simulink model "AMR_Testing"  (R2023b)
settings: Solver=FixedStepAuto  StartTime=0.0  StopTime=inf  FixedStep=1e-3  RelTol=1e-3
model workspace (MAT data in the model file):
  mdlWSDbList = ["C:\Users\matlab.cut\Desktop\AMR\canbus_files\tramontina_database_mobotic.dbc" "C:\Users\matlab.cut\Desktop\AMR\canbus_files\tramontina_database_nvidia.dbc" "C:\Users\matlab.cut\Desktop\AMR\canbus_files\tramontina_database_sick_modbus.dbc" "C:\Users\matlab.cut\Desktop\AMR\canbus_files\tramontina_database_xsens.dbc" "tramontina_database_curtis.dbc"]
  min_motor_rpm = 30
  vehicle_track = 877
  vehicle_wheelbase = 2367
  wheel_diameter = 360
  wheel_radius = 180
undefined symbols (not defined in the file or in its folder): Down, Pull
libraries: speedgoatlib_IO60X_IO69X x12, tramontina_database_curtislib x11, tramontina_database_nvidialib x5, simulink x4, tramontina_database_xsenslib x3, speedgoatlib_IO691 x2, simulink_extras x1, tramontina_database_sick_modbuslib x1, canmsglib x1
(part 1 of 2)
settings Model: SimulationMode=external  ExtModeEnableFloating=off  Creator=matlab.cut  LastModifiedBy=matlab.cut
settings SolverCC: ConcurrentTasks=on  PositivePriorityOrder=on
settings OptimizationCC: BlockReduction=off  OptimizeBlockIOStorage=off
settings DebuggingCC: TasksWithSamePriorityMsg=none
settings HardwareCC: ProdBitPerLong=64  ProdLongLongMode=on  ProdHWDeviceType=Intel->x86-64 (Linux 64)
settings ModelReferenceCC: ModelReferenceNumInstancesAllowed=Single
settings RTWCC: Description=Simulink Real-Time  SystemTargetFile=slrealtime.tlc  TemplateMakefile=slrealtime_default_tmf  Toolchain=Simulink Real-Time Toolchain  BuildConfiguration=Faster Runs  CodeExecutionProfiling=on  TargetLang=C++
settings CodeAppCC: MaxIdLength=127

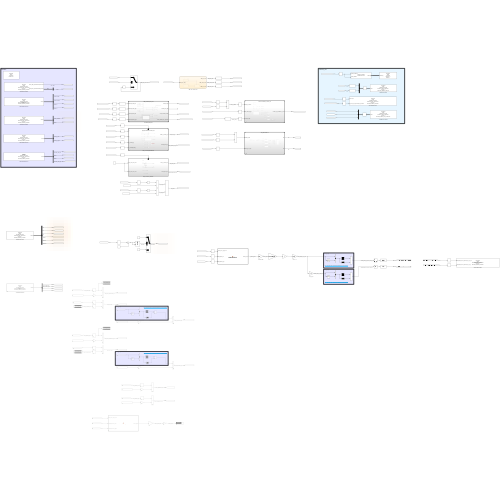
[thumbnail: Simulink's stored preview of the top-level diagram]
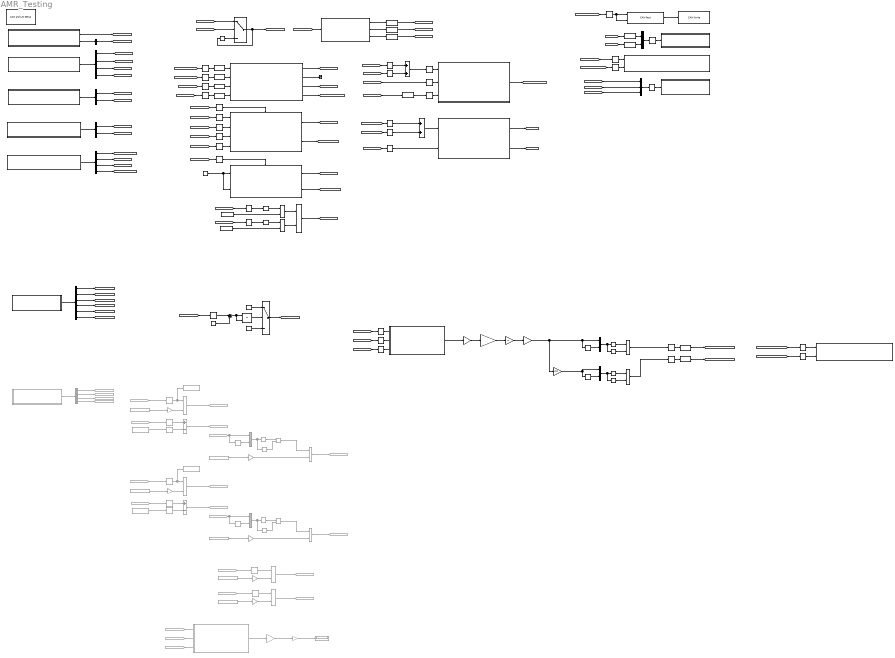
== system AMR_Testing ==
  note: moving_avg
  note: interface_out
  note: REF ->> https://www.youtube.com/watch?v=BV3H-0wlcSs&ab_channel=EmbeddedRoom
  note: REF ->> https://www.youtube.com/watch?v=BV3H-0wlcSs&ab_channel=EmbeddedRoom
  note: moving_avg
  note: REF ->> https://www.youtube.com/watch?v=BV3H-0wlcSs&ab_channel=EmbeddedRoom
  note: moving_avg
  note: REF ->> https://www.youtube.com/watch?v=BV3H-0wlcSs&ab_channel=EmbeddedRoom
  note: moving_avg
  note: interface
  AMR_ControlUnit_AutoMode : Subsystem  TreatAsAtomicUnit=on
  AMR_ControlUnit_ManualMode : ModelReference  ModelNameDialog=AMR_ManualModeControlUnit_23b.slx  SimulationMode=Normal  ModelReferenceVersion=1.27  EnablePortName=Enable  EnablePortStatesWhenEnabling=held
  AMR_oper_mode_chart : Stateflow chart  TreatAsAtomicUnit=on
  AND : Logic  AllPortsSameDT=off  OutDataTypeStr=boolean
  Abs : Abs  SaturateOnIntegerOverflow=off
  Abs3 : Abs  SaturateOnIntegerOverflow=off
  Add1 : Sum
  Add2 : Sum
  Bus Creator1 : BusCreator  Inputs=2
  Bus Creator2 : BusCreator  Inputs=3
  Bus Selector10 : BusSelector  OutputSignals=ID422_curtis_feedback_message_left.motor_rpm_left,ID423_curtis_feedback_message_right.motor_rpm_right
  Bus Selector11 : BusSelector  OutputSignals=Status  OutputAsBus=on
  Bus Selector12 : BusSelector  OutputSignals=ID368_joystick_axes.joystick_throttle,ID368_joystick_axes.joystick_direction,ID369_joystick_buttons.button_5,ID369_joystick_buttons.button_6
  Bus Selector13 : BusSelector  OutputSignals=ID1830_controller_status_left.controller_mode_left,ID1830_controller_status_left.MessageStatus.Status,ID1831_controller_status_right.MessageStatus.Status,ID1831_controller_status_right.controller_mode_right
  Bus Selector5 : BusSelector  OutputSignals=ID49_DeltaV.X,ID49_DeltaV.Y,ID49_DeltaV.Z,ID49_DeltaV.MessageStatus.Status,ID17_StatusWord.GNSSfix,ID17_StatusWord.RtkStatus
  Bus Selector6 : BusSelector  Commented=on  OutputSignals=ID934_curtis_encoder_left.rotor_position_left,ID935_curtis_encoder_right.rotor_position_rigth,ID934_curtis_encoder_left.MessageStatus.Status,ID935_curtis_encoder_right.MessageStatus.Status
  Bus Selector7 : BusSelector  Commented=on  OutputSignals=ID934_curtis_encoder_left.rotor_position_left,ID935_curtis_encoder_right.rotor_position_rigth,ID934_curtis_encoder_left.MessageStatus.Status,ID935_curtis_encoder_right.MessageStatus.Status
  Bus Selector9 : BusSelector  OutputSignals=ID288_mobotic_feedback_pos.position_feedback,ID288_mobotic_feedback_pos.MessageStatus.Status
  "CAN DB Parser Read " : Subsystem
      settings: OpenFcn=sg_can.OpenFcnRead;
      mask Help: eval('sg.utils.help.show(''io_main/refentry_ref_can_ofa_parsing_read'');')
      mask Display: disp('Speedgoat\nIO691\nCAN DB Parser Read\nModule ID: IO691 - Module ID 1\nChannel:  1\ntramontina_database_xsens.dbc ');
  CAN DB Parser Read 10 : Subsystem
      settings: OpenFcn=sg_can.OpenFcnRead;
      mask Help: eval('sg.utils.help.show(''io_main/refentry_ref_can_ofa_parsing_read'');')
      mask Display: disp('Speedgoat\nIO691\nCAN DB Parser Read\nModule ID: IO691 - Module ID 1\nChannel:  1\ntramontina_database_curtis.dbc ');
  CAN DB Parser Read 11 : Subsystem
      settings: OpenFcn=sg_can.OpenFcnRead;
      mask Help: eval('sg.utils.help.show(''io_main/refentry_ref_can_ofa_parsing_read'');')
      mask Display: disp('Speedgoat\nIO691\nCAN DB Parser Read\nModule ID: IO691 - Module ID 1\nChannel:  1\ntramontina_database_curtis.dbc ');
  CAN DB Parser Read 12 : Subsystem
      settings: OpenFcn=sg_can.OpenFcnRead;
      mask Help: eval('sg.utils.help.show(''io_main/refentry_ref_can_ofa_parsing_read'');')
      mask Display: disp('Speedgoat\nIO691\nCAN DB Parser Read\nModule ID: IO691 - Module ID 1\nChannel:  1\ntramontina_database_nvidia.dbc ');
  CAN DB Parser Read 6 : Subsystem  Commented=on
      settings: OpenFcn=sg_can.OpenFcnRead;
      mask Help: eval('sg.utils.help.show(''io_main/refentry_ref_can_ofa_parsing_read'');')
      mask Display: disp('Speedgoat\nIO691\nCAN DB Parser Read\nModule ID: IO691 - Module ID 1\nChannel:  1\ntramontina_database_curtis.dbc ');
  CAN DB Parser Read 7 : Subsystem  Commented=on
      settings: OpenFcn=sg_can.OpenFcnRead;
      mask Help: eval('sg.utils.help.show(''io_main/refentry_ref_can_ofa_parsing_read'');')
      mask Display: disp('Speedgoat\nIO691\nCAN DB Parser Read\nModule ID: IO691 - Module ID 1\nChannel:  1\ntramontina_database_curtis.dbc ');
  CAN DB Parser Read 8 : Subsystem
      settings: OpenFcn=sg_can.OpenFcnRead;
      mask Help: eval('sg.utils.help.show(''io_main/refentry_ref_can_ofa_parsing_read'');')
      mask Display: disp('Speedgoat\nIO691\nCAN DB Parser Read\nModule ID: IO691 - Module ID 1\nChannel:  1\ntramontina_database_nvidia.dbc ');
  CAN DB Parser Read 9 : Subsystem
      settings: OpenFcn=sg_can.OpenFcnRead;
      mask Help: eval('sg.utils.help.show(''io_main/refentry_ref_can_ofa_parsing_read'');')
      mask Display: disp('Speedgoat\nIO691\nCAN DB Parser Read\nModule ID: IO691 - Module ID 1\nChannel:  1\ntramontina_database_nvidia.dbc ');
  "CAN DB Parser Write " : Subsystem
      settings: OpenFcn=sg_can.OpenFcnWrite;
      mask Help: eval('sg.utils.help.show(''io_main/refentry_ref_can_ofa_parsing_write'');')
      mask Display: disp('Speedgoat\nIO691\nCAN DB Parser Write\nModule ID: IO691 - Module ID 1\nChannel:  1\ntramontina_database_curtis.dbc ');
  CAN DB Parser Write 1 : Subsystem
      settings: OpenFcn=sg_can.OpenFcnWrite;
      mask Help: eval('sg.utils.help.show(''io_main/refentry_ref_can_ofa_parsing_write'');')
      mask Display: disp('Speedgoat\nIO691\nCAN DB Parser Write\nModule ID: IO691 - Module ID 1\nChannel:  1\ntramontina_database_curtis.dbc ');
  CAN DB Parser Write 2 : Subsystem
      settings: OpenFcn=sg_can.OpenFcnWrite;
      mask Help: eval('sg.utils.help.show(''io_main/refentry_ref_can_ofa_parsing_write'');')
      mask Display: disp('Speedgoat\nIO691\nCAN DB Parser Write\nModule ID: IO691 - Module ID 1\nChannel:  1\ntramontina_database_sick_modbus.dbc ');
  CAN DB Parser Write 3 : Subsystem
      settings: OpenFcn=sg_can.OpenFcnWrite;
      mask Help: eval('sg.utils.help.show(''io_main/refentry_ref_can_ofa_parsing_write'');')
      mask Display: disp('Speedgoat\nIO691\nCAN DB Parser Write\nModule ID: IO691 - Module ID 1\nChannel:  1\ntramontina_database_nvidia.dbc ');
  CAN Pack1 : canmsglib/CAN Pack  MsgList=(none)  MsgName=CAN Msg  MsgIDType=Standard (11-bit identifier)  MsgIdentifier=0x120  MsgLength=8  Remote=off  ApplyMinMax=off  BusOutput=on  SignalInfo={ 'position_feedback', '0', '32', 'LE', 'signed', 'Standard', '0', '1', '0', '-inf', 'inf'; 'pulse_feedback', '32', '32', 'LE', 'signed', 'Standard', '0', '1', '0', '-Inf', 'Inf' }
      settings: DataFormat=manually specified signals
  "CAN Write " : speedgoatlib_IO691/CAN Write   moduleType=IO691  id=1  channel=1  canType=CAN (HS)  messageType=CAN (HS)  useBusIn=on  numOfMsg=1  enableInput=off  enableStatusPort=off  ts=20e-3  initValues=[691 1 0.02 0 1 1 0 1 0 1]
      settings: SourceProductName=Simulink Real-Time: Speedgoat I/O Blockset
  CAN and LIN Setup 1 : speedgoatlib_IO691/CAN and LIN Setup   moduleInitValues="[691    1    1   -1   -1]"  id=1  moduleType=IO691  pciSlot=-1  canChn1=CAN (HS)  canChn2=Disabled  canChn3=Disabled  canChn4=Disabled  linChn1=Disabled  linChn2=Disabled  canInitStructArray=[]  canTermStructArray=[]  gpioChnx=Disabled  canChn1InitValues="[2   2   8   1  16   3  19   2   2   5   2   0]"  arbBdrChn1=500 kBaud  clockDividerChn1=Enable  arbManBdrChn1=[8,1,16,3]  fdBdrChn1=5.0 MBaud  fdManBdrChn1=[2,2,5,2]  termResistor1=off  canChn2InitValues="[1   0   2   8  31   8  19   2   2   5   2   0]"  arbBdrChn2=1.0 MBaud  clockDividerChn2=Enable  arbManBdrChn2=[2,8,31,8]  fdBdrChn2=5.0 MBaud  fdManBdrChn2=[2,2,5,2]  termResistor2=off  canChn3InitValues="[1   0   2   8  31   8  19   2   2   5   2   0]"  arbBdrChn3=1.0 MBaud  clockDividerChn3=Enable  arbManBdrChn3=[2,8,31,8]  fdBdrChn3=5.0 MBaud  fdManBdrChn3=[2,2,5,2]  termResistor3=off  canChn4InitValues="[1   0   2   8  31   8  19   2   2   5   2   0]"  arbBdrChn4=1.0 MBaud  clockDividerChn4=Enable  arbManBdrChn4=[2,8,31,8]  fdBdrChn4=5.0 MBaud  fdManBdrChn4=[2,2,5,2]  termResistor4=off  linChn1InitValues="[0  9600]"  linBtrChn1=9600  linChn2InitValues="[0  9600]"  linBtrChn2=9600  doInitTermStruct="[0  5  0  0  0]"  parDoChannels=[1 2]  parDoVoltage=5  parDoInitValues=0  parDoReset=1  parNumOfDoS=0  parDiChannels=[3 4]  parDiVoltage=5  parDiPull=Pull-Down
      settings: LibrarySourceBlock=speedgoatlib_IO602_IO691/CAN and LIN Setup
  Cast : DataTypeConversion  OutDataTypeStr=double  SaturateOnIntegerOverflow=off  RndMeth=Floor
  Cast1 : DataTypeConversion  OutDataTypeStr=uint8  SaturateOnIntegerOverflow=off  RndMeth=Floor
  Cast10 : DataTypeConversion  OutDataTypeStr=single  SaturateOnIntegerOverflow=off  RndMeth=Floor
  Cast12 : DataTypeConversion  OutDataTypeStr=single  SaturateOnIntegerOverflow=off  RndMeth=Floor
  Cast{2..3,6..9} (6 alike) : DataTypeConversion  OutDataTypeStr=boolean  SaturateOnIntegerOverflow=off  RndMeth=Floor
  Cast4 : DataTypeConversion  OutDataTypeStr=uint8  SaturateOnIntegerOverflow=off  RndMeth=Floor
  Cast5 : DataTypeConversion  OutDataTypeStr=double  SaturateOnIntegerOverflow=off  RndMeth=Floor
  Constant : Constant
  Constant1 : Constant  Value=min_motor_rpm
  Constant10 : Constant
  Constant{2..4,6..7,11} (6 alike) : Constant  Commented=on  Value=wheel_diameter
  Constant5 : Constant  Value=min_motor_rpm
  Constant8 : Constant
  Constant9 : Constant  Value=0
  Data Store Read : DataStoreRead  Commented=on  DataStoreName=rotor_positon_right  DataStoreElements=rotor_positon_right  IndexOptions=Index vector (dialog)  Indices=1  OutputSizes=1
  Data Store Read1 : DataStoreRead  Commented=on  DataStoreName=rotor_positon_left  DataStoreElements=rotor_positon_left  IndexOptions=Index vector (dialog)  Indices=1  OutputSizes=1
  Data Store Write : DataStoreWrite  Commented=on  DataStoreName=rotor_positon_left  DataStoreElements=rotor_positon_left  IndexOptions=Index vector (dialog)  Indices=1  OutputSizes=1
  Data Store Write1 : DataStoreWrite  Commented=on  DataStoreName=rotor_positon_right  DataStoreElements=rotor_positon_right  IndexOptions=Index vector (dialog)  Indices=1  OutputSizes=1
  Display3 : Display  Commented=on
  Divide{1..6} (6 alike) : Product  Commented=on  Inputs=**
  Equal3 : RelationalOperator  Operator=>  OutDataTypeStr=boolean  RndMeth=Simplest  InputSameDT=off
  Equal4 : RelationalOperator  Operator=>  OutDataTypeStr=boolean  RndMeth=Simplest  InputSameDT=off
  From34 : From  Commented=on  GotoTag=rotor_positon_left
  From36 : From  Commented=on  GotoTag=rotor_positon_left
  From37 : From  Commented=on  GotoTag=rotor_positon_right
  From38 : From  Commented=on  GotoTag=linear_disp_left
  From39 : From  Commented=on  GotoTag=linear_disp_right
  From40 : From  Commented=on  GotoTag=steering_unit_pos
  From41 : From  Commented=on  GotoTag=delta_revol_left
  From42 : From  Commented=on  GotoTag=rotor_positon_right
  From43 : From  Commented=on  GotoTag=rotor_positon_right
  From44 : From  Commented=on  GotoTag=delta_revol_right
  From46 : From  Commented=on  GotoTag=rotor_positon_left
  Gain{1,4..7,9} (6 alike) : Gain  Commented=on  Gain=pi
  Gain11 : Gain  Gain=pi
  Gain2 : Gain  Commented=on  Gain=5
  Gain3 : Gain  Commented=on  Gain=1/1000
  Gain8 : Gain  Gain=wheel_diameter
  Goto15 : Goto  Commented=on  GotoTag=rotor_positon_right
  Goto29 : Goto  Commented=on  GotoTag=rotor_positon_left
  Goto31 : Goto  Commented=on  GotoTag=rotor_status_left
  Goto32 : Goto  Commented=on  GotoTag=linear_disp_left
  Goto39 : Goto  Commented=on  GotoTag=rotor_positon_right
  Goto40 : Goto  Commented=on  GotoTag=rotor_status_right
  Goto42 : Goto  Commented=on  GotoTag=total_linear_disp_left
  Goto43 : Goto  Commented=on  GotoTag=linear_disp_right
  Goto44 : Goto  Commented=on  GotoTag=delta_revol_left
  Goto45 : Goto  Commented=on  GotoTag=linear_disp_right
  Goto46 : Goto  Commented=on  GotoTag=total_linear_disp_right
  Goto47 : Goto  Commented=on  GotoTag=delta_revol_right
  Goto48 : Goto  Commented=on  GotoTag=rotor_positon_left
  Goto49 : Goto  Commented=on  GotoTag=linear_disp_left
  Goto50 : Goto  Commented=on  GotoTag=rotor_status_left
  Goto51 : Goto  Commented=on  GotoTag=rotor_status_right
  Integrator1 : Integrator  ExternalReset=either  UpperSaturationLimit=1  LowerSaturationLimit=0  WrappedStateUpperValue=30  WrappedStateLowerValue=0
  MATLAB Function : MATLAB Function  Commented=on  TreatAsAtomicUnit=on
  MATLAB Function1 : MATLAB Function  TreatAsAtomicUnit=on
  Memory : Memory  InheritSampleTime=on
  Model : ModelReference  ModelNameDialog=AMR_differentialDrive.slx  SimulationMode=Normal  ModelReferenceVersion=1.11
  Model1 : ModelReference  ModelNameDialog=MotorControllerDrive_mobotic_23b.slx  SimulationMode=Normal  ModelReferenceVersion=1.56
  MotorStartupSequence : ModelReference  ModelNameDialog=AMR_MotorStartupUnit_23b.slx  SimulationMode=Normal  ModelReferenceVersion=1.19
  Product : Product  Commented=on  Inputs=*/
  Product1 : Product  Commented=on  Inputs=*/
  Product2 : Product  Inputs=*/
  Product3 : Product  Inputs=*/
  Rate Transition{1..29,32,38,40..41} (33 alike) : RateTransition
  Rate Transition{30..31,33..37,39} (8 alike) : RateTransition  Commented=on
  Subtract : Sum  Commented=on  Inputs=+-
  Subtract1 : Sum  Commented=on  Inputs=+-
  Sum : Sum  Inputs=|+-
  Sum of Elements : Sum  Commented=on  Inputs=+
  Sum of Elements1 : Sum  Commented=on  Inputs=+
  Sum of Elements2 : Sum  Inputs=+
  Sum of Elements3 : Sum  Inputs=+
  Switch : Switch  Criteria=u2 > Threshold  SaturateOnIntegerOverflow=off  InputSameDT=off
  Switch1 : Switch  Criteria=u2 > Threshold  Threshold=30  SaturateOnIntegerOverflow=off  InputSameDT=off
  Tapped Delay : simulink/Discrete/Tapped Delay  Commented=on  vinit=0  samptime=-1  NumDelays=3  DelayOrder=Oldest  includeCurrent=off
  Tapped Delay1 : simulink/Discrete/Tapped Delay  Commented=on  vinit=0  samptime=-1  NumDelays=3  DelayOrder=Oldest  includeCurrent=off
  Tapped Delay2 : simulink/Discrete/Tapped Delay  vinit=0  samptime=-1  NumDelays=9  DelayOrder=Oldest  includeCurrent=off
  Tapped Delay3 : simulink/Discrete/Tapped Delay  vinit=0  samptime=-1  NumDelays=9  DelayOrder=Oldest  includeCurrent=off
  Terminator : Terminator
  Vector Concatenate : Concatenate  Commented=on
  Vector Concatenate1 : Concatenate  Commented=on
  Vector Concatenate2 : Concatenate
  Vector Concatenate3 : Concatenate
  Width : Width  Commented=on
  Width1 : Width  Commented=on
  Width2 : Width
  Width3 : Width
  gearbox_ratio : Gain  Gain=1/40.61
  mm_to_m : Gain  Gain=1/1000
  mm_to_m1 : Gain  Gain=1/60
  wires:
  Switch/1 -> [AMR_oper_mode], Memory/1  "AMR_oper_mode"
  Memory/1 -> Switch/3
  [oper_mode] -> Switch/1
  [oper_mode_status] -> Switch/2
  [yj] -> Rate Transition2/1
  [joy_maxspeed_flag] -> Rate Transition4/1
  [xj] -> Rate Transition1/1
  [joy_boost_flag] -> Rate Transition3/1
  AMR_ControlUnit_ManualMode/1 -> [theta_from_joy]  "theta_from_joy"
  [steering_unit_pos] -> Rate Transition5/1
  AMR_ControlUnit_AutoMode/1(theta_to_mobotic_auto) -> [theta_from_auto]  "theta_from_auto"
  AMR_ControlUnit_AutoMode/2(throttle_speed_auto) -> [throttle_speed_from_auto]  "throttle_speed_from_auto"
  Rate Transition1/1 -> AMR_ControlUnit_ManualMode/1
  Rate Transition2/1 -> AMR_ControlUnit_ManualMode/2
  Rate Transition3/1 -> AMR_ControlUnit_ManualMode/3
  Rate Transition4/1 -> AMR_ControlUnit_ManualMode/4
  [theta_from_joy] -> Rate Transition7/1
  [steering_unit_ready] -> Cast3/1
  Add1/1 -> Rate Transition14/1  "theta_to_mobotic"
  Rate Transition9/1 -> AMR_ControlUnit_AutoMode/Enable
  CAN Pack1/1 -> "CAN Write "/1
  [steering_unit_theta_position] -> Rate Transition10/1
  Model1/1 -> [steering_unit_theta_position]
  Rate Transition10/1 -> CAN Pack1/2, CAN Pack1/1
  [theta_from_auto] -> Rate Transition11/1
  Rate Transition7/1 -> Add1/1
  Rate Transition11/1 -> Add1/2
  Cast3/1 -> Rate Transition19/1  "mobotic_ready"
  [hold_theta] -> Rate Transition18/1
  AMR_ControlUnit_ManualMode/2 -> [throttle_speed_from_joy]  "throttle_speed_from_joy"
  [lws] -> Cast/1  "lws"
  [rws] -> Cast5/1  "rws"
  Cast/1 -> Bus Creator1/1
  Bus Creator1/1 -> Rate Transition15/1
  Cast5/1 -> Bus Creator1/2
  Rate Transition15/1 -> "CAN DB Parser Write "/1(CAN Tx)
  [AMR_oper_mode] -> AMR_oper_mode_chart/1(AMR_oper_mode)
  [AMR_manual_mode] -> Rate Transition16/1
  AMR_oper_mode_chart/3(AMR_auto_mode) -> Cast7/1  "AMR_auto_mode"
  AMR_oper_mode_chart/1(AMR_idle_mode) -> Cast8/1  "AMR_idle_mode"
  AMR_oper_mode_chart/2(AMR_manual_mode) -> Cast6/1  "AMR_manual_mode"
  Rate Transition16/1 -> AMR_ControlUnit_ManualMode/Enable
  Cast6/1 -> [AMR_manual_mode]
  Cast7/1 -> [AMR_auto_mode]
  Cast8/1 -> [AMR_idle_mode]
  [AMR_auto_mode] -> Rate Transition9/1
  Model/1 -> [lws]  "lws"
  Model/2 -> [rws]  "rws"
  AND/1 -> [hold_theta]  "hold_theta"
  [motor_rpm_right] -> Rate Transition13/1
  Abs/1 -> Equal3/1
  Constant5/1 -> Equal3/2
  Equal3/1 -> AND/1  "min_vel_left"
  Constant1/1 -> Equal4/2
  Equal4/1 -> AND/2  "min_vel_right"
  [motor_rpm_left] -> Rate Transition17/1
  Abs3/1 -> Equal4/1
  Rate Transition17/1 -> Abs/1
  Rate Transition13/1 -> Abs3/1
  Constant/1 -> AMR_ControlUnit_AutoMode/2(input2_from_auto_mode), AMR_ControlUnit_AutoMode/1(input1_from_auto_mode)
  Rate Transition12/1 -> Add2/2
  Add2/1 -> Model/1
  Rate Transition8/1 -> Add2/1
  [throttle_speed_from_auto] -> Rate Transition12/1
  [throttle_speed_from_joy] -> Rate Transition8/1
  Rate Transition5/1 -> Model/2
  MotorStartupSequence/2 -> Terminator/1
  MotorStartupSequence/1 -> [steering_unit_ready]
  [controller_enable_flag] -> Rate Transition24/1
  [curtis_controller_into_operation] -> Rate Transition6/1
  Rate Transition6/1 -> CAN DB Parser Write 1/2(ID0_curtis_input_operational.pre_operational)
  Rate Transition14/1 -> Model1/1
  Rate Transition18/1 -> Model1/2
  Rate Transition19/1 -> Model1/3
  Rate Transition24/1 -> CAN DB Parser Write 1/1(Enable Input)
  MotorStartupSequence/3 -> [controller_enable_flag]
  MotorStartupSequence/4 -> [curtis_controller_into_operation]
  Rate Transition21/1 -> Cast4/1
  [curtis_controller_mode_right] -> Rate Transition20/1
  Rate Transition22/1 -> Cast2/1
  Rate Transition23/1 -> Cast9/1
  Cast4/1 -> MotorStartupSequence/1
  Cast1/1 -> MotorStartupSequence/2
  Cast2/1 -> MotorStartupSequence/3
  Cast9/1 -> MotorStartupSequence/4
  Rate Transition20/1 -> Cast1/1
  [curtis_controller_mode_left] -> Rate Transition21/1
  [curtis_status_left] -> Rate Transition22/1
  [curtis_status_right] -> Rate Transition23/1
  [AMR_idle_mode] -> Bus Creator2/1
  [AMR_manual_mode] -> Bus Creator2/2
  [AMR_auto_mode] -> Bus Creator2/3
  Bus Creator2/1 -> Rate Transition25/1
  Rate Transition25/1 -> CAN DB Parser Write 2/1(CAN Tx)
  Bus Selector5/4 -> [deltaV_status]  "<Status>"
  Bus Selector5/3 -> [z]  "<Z>"
  "CAN DB Parser Read "/1(CAN Rx) -> Bus Selector5/1
  Bus Selector5/5 -> [GPS_GNSSfix]  "<GNSSfix>"
  Bus Selector5/6 -> [GPS_RTKstatus]  "<RtkStatus>"
  Bus Selector5/2 -> [y]  "<Y>"
  Bus Selector5/1 -> [x]  "<X>"
  [GPS_RTKstatus] -> Rate Transition29/1
  Constant10/1 -> Sum/2
  Sum/1 -> Integrator1/2, Integrator1/1  "diff"
  Constant8/1 -> Switch1/1
  Switch1/1 -> [GPS_rtk_trustness]  "rtk_trustness"
  Constant9/1 -> Switch1/3
  Integrator1/1 -> Switch1/2  "integrator"
  Rate Transition29/1 -> Sum/1
  Bus Selector6/4 -> Goto40/1  "<Status>"
  Bus Selector6/1 -> Goto29/1  "<rotor_position_left>"
  Bus Selector6/2 -> Goto15/1  "<rotor_position_rigth>"
  CAN DB Parser Read 6/1(CAN Rx) -> Bus Selector6/1
  Bus Selector6/3 -> Goto31/1  "<Status>"
  Divide3/1 -> Goto42/1  "total_linear_displacement_left"
  Constant2/1 -> Gain4/1
  Rate Transition31/1 -> Divide3/1, Data Store Write/1
  Constant3/1 -> Gain1/1
  Divide1/1 -> Goto43/1  "linear_displacement_right"
  From37/1 -> Rate Transition33/1  "rotor_position_right"
  Rate Transition33/1 -> Divide1/1
  From38/1 -> MATLAB Function/2(Total_Displacement_Left)
  From39/1 -> MATLAB Function/3(Total_Displacement_Right)
  Gain2/1 -> Display3/1  "vehicle_speed"
  From40/1 -> MATLAB Function/1(Actual_Curve_Angle_Front)
  Gain3/1 -> Gain2/1  "vehicle_speed_ratio"
  MATLAB Function/1(vehicle_speed) -> Gain3/1
  From34/1 -> Rate Transition31/1  "rotor_position_left"
  From36/1 -> Rate Transition30/1
  Subtract/1 -> Goto44/1  "delta_revol_left"
  Gain4/1 -> Divide3/2
  Constant4/1 -> Gain5/1
  Gain5/1 -> Divide2/2
  Divide2/1 -> Goto32/1  "linear_displacement_left"
  Rate Transition30/1 -> Subtract/1
  Data Store Read1/1 -> Rate Transition34/1  "rotor_pos_memo_left"
  Rate Transition34/1 -> Subtract/2
  Vector Concatenate/1 -> Sum of Elements/1, Width/1
  Product/1 -> Divide2/1
  Sum of Elements/1 -> Product/1
  Width/1 -> Product/2
  Tapped Delay/1 -> Vector Concatenate/2
  From41/1 -> Tapped Delay/1, Vector Concatenate/1
  Sum of Elements1/1 -> Product1/1
  Width1/1 -> Product1/2
  Vector Concatenate1/1 -> Sum of Elements1/1, Width1/1
  Data Store Read/1 -> Rate Transition37/1  "rotor_pos_memo_right"
  Rate Transition37/1 -> Subtract1/2
  From44/1 -> Tapped Delay1/1, Vector Concatenate1/1
  Rate Transition35/1 -> Subtract1/1
  Product1/1 -> Divide4/1
  Gain7/1 -> Divide4/2
  Constant7/1 -> Gain7/1
  Subtract1/1 -> Goto47/1  "delta_revol_right"
  Rate Transition36/1 -> Divide5/1, Data Store Write1/1
  Constant6/1 -> Gain6/1
  From43/1 -> Rate Transition35/1
  Gain6/1 -> Divide5/2
  Divide5/1 -> Goto46/1  "total_linear_displacement_right"
  Divide4/1 -> Goto45/1  "linear_displacement_right"
  Tapped Delay1/1 -> Vector Concatenate1/2
  From42/1 -> Rate Transition36/1  "rotor_position_right"
  Rate Transition39/1 -> Divide6/1
  From46/1 -> Rate Transition39/1  "rotor_position_left"
  Divide6/1 -> Goto49/1  "linear_displacement_left"
  Constant11/1 -> Gain9/1
  Gain9/1 -> Divide6/2
  Gain1/1 -> Divide1/2
  [steering_unit_pos] -> Rate Transition38/1
  Gain8/1 -> Gain11/1
  gearbox_ratio/1 -> Gain8/1  "wheel_speed"
  [motor_rpm_left] -> Rate Transition40/1
  [motor_rpm_right] -> Rate Transition41/1
  MATLAB Function1/1(Vehicle_Speed) -> gearbox_ratio/1  "gearbox_speed"
  Gain11/1 -> mm_to_m/1
  Rate Transition38/1 -> MATLAB Function1/1(Actual_Curve_Angle_Front)
  Rate Transition40/1 -> MATLAB Function1/2(RPM_Speed_Left)
  Rate Transition41/1 -> MATLAB Function1/3(RPM_Speed_Right)
  mm_to_m/1 -> Tapped Delay2/1, Vector Concatenate2/1, mm_to_m1/1  "vehicle_speed_m_per_min"
  Product2/1 -> Rate Transition26/1  "vehicle_speed_m_per_min_mov_avg"
  Vector Concatenate2/1 -> Sum of Elements2/1, Width2/1
  Tapped Delay2/1 -> Vector Concatenate2/2
  Sum of Elements2/1 -> Product2/1
  Width2/1 -> Product2/2
  Bus Selector7/3 -> Goto50/1  "<Status>"
  CAN DB Parser Read 7/1(CAN Rx) -> Bus Selector7/1
  Bus Selector7/2 -> Goto39/1  "<rotor_position_rigth>"
  Bus Selector7/1 -> Goto48/1  "<rotor_position_left>"
  Bus Selector7/4 -> Goto51/1  "<Status>"
  Width3/1 -> Product3/2
  Sum of Elements3/1 -> Product3/1
  Tapped Delay3/1 -> Vector Concatenate3/2
  Vector Concatenate3/1 -> Width3/1, Sum of Elements3/1
  mm_to_m1/1 -> Vector Concatenate3/1, Tapped Delay3/1  "vehicle_speed_m_per_sec"
  Product3/1 -> Rate Transition27/1  "vehicle_speed_m_per_sec_mov_avg"
  Rate Transition26/1 -> Cast10/1
  Rate Transition27/1 -> Cast12/1
  Cast10/1 -> [AMR_speed_to_CAN_m_per_min]
  Cast12/1 -> [AMR_speed_to_CAN_m_per_sec]
  [AMR_speed_to_CAN_m_per_min] -> Rate Transition28/1
  Rate Transition28/1 -> CAN DB Parser Write 3/1(ID290_AMR_vehicle_speed.speed_m_per_min)
  Rate Transition32/1 -> CAN DB Parser Write 3/2(ID290_AMR_vehicle_speed.speed_m_per_s)
  [AMR_speed_to_CAN_m_per_sec] -> Rate Transition32/1
  CAN DB Parser Read 8/1(ID343_AMR_OperationMode.OperationMode) -> [oper_mode]  "oper_mode"
  CAN DB Parser Read 12/1(CAN Rx) -> Bus Selector12/1
  CAN DB Parser Read 9/1(CAN Rx) -> Bus Selector9/1
  Bus Selector10/1 -> [motor_rpm_left]  "<motor_rpm_left>"
  CAN DB Parser Read 11/1(CAN Rx) -> Bus Selector13/1
  Bus Selector12/1 -> [xj]  "<joystick_throttle>"
  Bus Selector12/3 -> [joy_boost_flag]  "<button_5>"
  Bus Selector11/1 -> [oper_mode_status]  "status"
  CAN DB Parser Read 8/2(ID343_AMR_OperationMode.MessageStatus) -> Bus Selector11/1  "status"
  CAN DB Parser Read 10/1(CAN Rx) -> Bus Selector10/1
  Bus Selector13/4 -> [curtis_controller_mode_right]  "<controller_mode_right>"
  Bus Selector9/2 -> [steering_unit_status]  "<Status>"
  Bus Selector13/3 -> [curtis_status_right]  "<Status>"
  Bus Selector13/2 -> [curtis_status_left]  "<Status>"
  Bus Selector9/1 -> [steering_unit_pos]  "<position_feedback>"
  Bus Selector12/2 -> [yj]  "<joystick_direction>"
  Bus Selector12/4 -> [joy_maxspeed_flag]  "<button_6>"
  Bus Selector13/1 -> [curtis_controller_mode_left]  "<controller_mode_left>"
  Bus Selector10/2 -> [motor_rpm_right]  "<motor_rpm_right>"

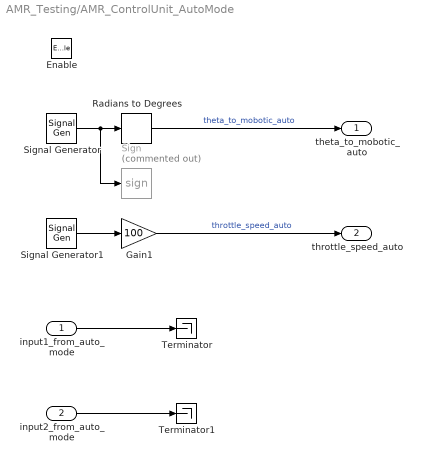
== system AMR_Testing/AMR_ControlUnit_AutoMode ==
  input1_from_auto_mode : Inport
  input2_from_auto_mode : Inport  Port=2
  Enable : EnablePort  OutDataTypeStr=boolean
  Gain1 : Gain  Gain=100
  Radians to Degrees : simulink_extras/Transformations/Radians to Degrees
  Sign : Signum  Commented=on
  Signal Generator : SignalGenerator  Amplitude=pi/6  Frequency=0.05
  Signal Generator1 : SignalGenerator  WaveForm=square  Frequency=0.01
  Terminator : Terminator
  Terminator1 : Terminator
  theta_to_mobotic_auto : Outport  OutputWhenDisabled=reset  InitialOutput=[0]
  throttle_speed_auto : Outport  Port=2  OutputWhenDisabled=reset  InitialOutput=[0]
  wires:
  Radians to Degrees/1 -> theta_to_mobotic_auto/1  "theta_to_mobotic_auto"
  Signal Generator/1 -> Sign/1, Radians to Degrees/1
  Gain1/1 -> throttle_speed_auto/1  "throttle_speed_auto"
  Signal Generator1/1 -> Gain1/1
  input1_from_auto_mode/1 -> Terminator/1
  input2_from_auto_mode/1 -> Terminator1/1

== system AMR_Testing/CAN DB Parser Read  ==
  ReadSubsystem : Subsystem
  UnpackSubsystem : Subsystem
  CAN Rx : Outport
  wires:
  ReadSubsystem/1(Raw_Rx) -> UnpackSubsystem/1(Unpack_In)
  ReadSubsystem/2(Status_Rx) -> UnpackSubsystem/2(Status Inport)
  UnpackSubsystem/1(Unpack_Out) -> CAN Rx/1

== system AMR_Testing/CAN DB Parser Read 10 ==
  ReadSubsystem : Subsystem
  UnpackSubsystem : Subsystem
  CAN Rx : Outport
  wires:
  ReadSubsystem/1(Raw_Rx) -> UnpackSubsystem/1(Unpack_In)
  ReadSubsystem/2(Status_Rx) -> UnpackSubsystem/2(Status Inport)
  UnpackSubsystem/1(Unpack_Out) -> CAN Rx/1

== system AMR_Testing/CAN DB Parser Read 11 ==
  ReadSubsystem : Subsystem
  UnpackSubsystem : Subsystem
  CAN Rx : Outport
  wires:
  ReadSubsystem/1(Raw_Rx) -> UnpackSubsystem/1(Unpack_In)
  ReadSubsystem/2(Status_Rx) -> UnpackSubsystem/2(Status Inport)
  UnpackSubsystem/1(Unpack_Out) -> CAN Rx/1

== system AMR_Testing/CAN DB Parser Read 12 ==
  ReadSubsystem : Subsystem
  UnpackSubsystem : Subsystem
  CAN Rx : Outport
  wires:
  ReadSubsystem/1(Raw_Rx) -> UnpackSubsystem/1(Unpack_In)
  ReadSubsystem/2(Status_Rx) -> UnpackSubsystem/2(Status Inport)
  UnpackSubsystem/1(Unpack_Out) -> CAN Rx/1

== system AMR_Testing/CAN DB Parser Read 6 ==
  ReadSubsystem : Subsystem
  UnpackSubsystem : Subsystem
  CAN Rx : Outport
  wires:
  ReadSubsystem/1(Raw_Rx) -> UnpackSubsystem/1(Unpack_In)
  ReadSubsystem/2(Status_Rx) -> UnpackSubsystem/2(Status Inport)
  UnpackSubsystem/1(Unpack_Out) -> CAN Rx/1

== system AMR_Testing/CAN DB Parser Read 7 ==
  ReadSubsystem : Subsystem
  UnpackSubsystem : Subsystem
  CAN Rx : Outport
  wires:
  UnpackSubsystem/1(Unpack_Out) -> CAN Rx/1
  ReadSubsystem/2(Status_Rx) -> UnpackSubsystem/2(Status Inport)
  ReadSubsystem/1(Raw_Rx) -> UnpackSubsystem/1(Unpack_In)

== system AMR_Testing/CAN DB Parser Read 8 ==
  ReadSubsystem : Subsystem
  SelectSignal_1_1 : BusSelector  OutputSignals=ID343_AMR_OperationMode.OperationMode
  SelectStatus_1 : BusSelector  OutputSignals=ID343_AMR_OperationMode.MessageStatus
  UnpackSubsystem : Subsystem
  ID343_AMR_OperationMode.OperationMode : Outport
  ID343_AMR_OperationMode.MessageStatus : Outport  Port=2
  wires:
  ReadSubsystem/1(Raw_Rx) -> UnpackSubsystem/1(Unpack_In)
  ReadSubsystem/2(Status_Rx) -> UnpackSubsystem/2(Status Inport)
  UnpackSubsystem/1(Unpack_Out) -> SelectSignal_1_1/1, SelectStatus_1/1
  SelectSignal_1_1/1 -> ID343_AMR_OperationMode.OperationMode/1  "<OperationMode>"
  SelectStatus_1/1 -> ID343_AMR_OperationMode.MessageStatus/1  "<MessageStatus>"

== system AMR_Testing/CAN DB Parser Read 9 ==
  ReadSubsystem : Subsystem
  UnpackSubsystem : Subsystem
  CAN Rx : Outport
  wires:
  ReadSubsystem/1(Raw_Rx) -> UnpackSubsystem/1(Unpack_In)
  ReadSubsystem/2(Status_Rx) -> UnpackSubsystem/2(Status Inport)
  UnpackSubsystem/1(Unpack_Out) -> CAN Rx/1

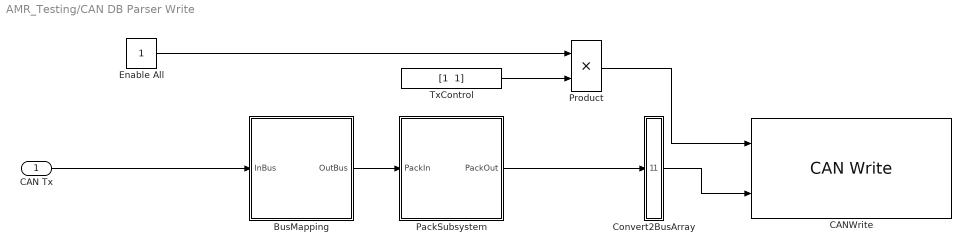
== system AMR_Testing/CAN DB Parser Write  ==
  CAN Tx : Inport
  BusMapping : Subsystem
  CANWrite : speedgoatlib_IO60X_IO69X/CAN/CAN Write   moduleType=IO691  id=1  channel=1  canType=CAN (HS)  messageType=CAN (HS)  useBusIn=on  numOfMsg=2  enableInput=on  enableStatusPort=off  ts=10e-3  initValues=[691 1 0.01 0 1 1 0 2 1 1]
  Convert2BusArray : Subsystem
  Enable All : Constant  OutDataTypeStr=boolean
  PackSubsystem : Subsystem
  Product : Product  OutDataTypeStr=uint32
  TxControl : Constant  Value="[1  1]"  OutDataTypeStr=uint32
  wires:
  PackSubsystem/1(PackOut) -> Convert2BusArray/1(InBus)
  Convert2BusArray/1(BusArrayOut) -> CANWrite/2
  Product/1 -> CANWrite/1
  TxControl/1 -> Product/2
  Enable All/1 -> Product/1
  CAN Tx/1 -> BusMapping/1(InBus)
  BusMapping/1(OutBus) -> PackSubsystem/1(PackIn)

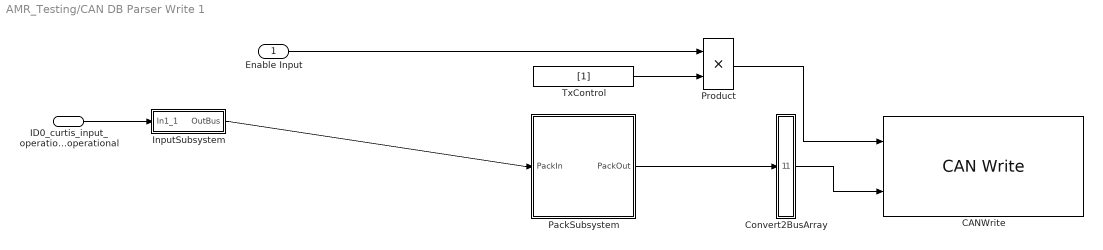
== system AMR_Testing/CAN DB Parser Write 1 ==
  Enable Input : Inport  OutDataTypeStr=boolean
  ID0_curtis_input_operational.pre_operational : Inport  Port=2
  CANWrite : speedgoatlib_IO60X_IO69X/CAN/CAN Write   moduleType=IO691  id=1  channel=1  canType=CAN (HS)  messageType=CAN (HS)  useBusIn=on  numOfMsg=1  enableInput=on  enableStatusPort=off  ts=500e-3  initValues=[691 1 0.5 0 1 1 0 1 1 1]
  Convert2BusArray : Subsystem
  InputSubsystem : Subsystem
  PackSubsystem : Subsystem
  Product : Product  OutDataTypeStr=uint32
  TxControl : Constant  Value=[1]  OutDataTypeStr=uint32
  wires:
  PackSubsystem/1(PackOut) -> Convert2BusArray/1(InBus)
  Convert2BusArray/1(BusArrayOut) -> CANWrite/2
  Product/1 -> CANWrite/1
  TxControl/1 -> Product/2
  Enable Input/1 -> Product/1
  ID0_curtis_input_operational.pre_operational/1 -> InputSubsystem/1(In1_1)
  InputSubsystem/1(OutBus) -> PackSubsystem/1(PackIn)

== system AMR_Testing/CAN DB Parser Write 2 ==
  CAN Tx : Inport
  BusMapping : Subsystem
  CANWrite : speedgoatlib_IO60X_IO69X/CAN/CAN Write   moduleType=IO691  id=1  channel=1  canType=CAN (HS)  messageType=CAN (HS)  useBusIn=on  numOfMsg=1  enableInput=on  enableStatusPort=off  ts=500e-3  initValues=[691 1 0.5 0 1 1 0 1 1 1]
  Convert2BusArray : Subsystem
  Enable All : Constant  OutDataTypeStr=boolean
  PackSubsystem : Subsystem
  Product : Product  OutDataTypeStr=uint32
  TxControl : Constant  Value=[1]  OutDataTypeStr=uint32
  wires:
  PackSubsystem/1(PackOut) -> Convert2BusArray/1(InBus)
  Convert2BusArray/1(BusArrayOut) -> CANWrite/2
  Product/1 -> CANWrite/1
  TxControl/1 -> Product/2
  Enable All/1 -> Product/1
  CAN Tx/1 -> BusMapping/1(InBus)
  BusMapping/1(OutBus) -> PackSubsystem/1(PackIn)

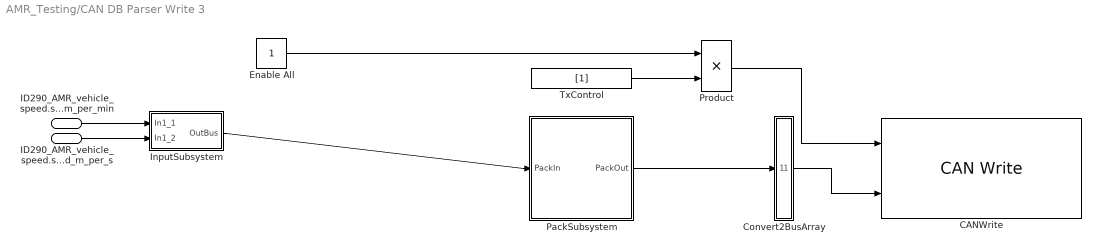
== system AMR_Testing/CAN DB Parser Write 3 ==
  ID290_AMR_vehicle_speed.speed_m_per_min : Inport
  ID290_AMR_vehicle_speed.speed_m_per_s : Inport  Port=2
  CANWrite : speedgoatlib_IO60X_IO69X/CAN/CAN Write   moduleType=IO691  id=1  channel=1  canType=CAN (HS)  messageType=CAN (HS)  useBusIn=on  numOfMsg=1  enableInput=on  enableStatusPort=off  ts=50e-3  initValues=[691 1 0.05 0 1 1 0 1 1 1]
  Convert2BusArray : Subsystem
  Enable All : Constant  OutDataTypeStr=boolean
  InputSubsystem : Subsystem
  PackSubsystem : Subsystem
  Product : Product  OutDataTypeStr=uint32
  TxControl : Constant  Value=[1]  OutDataTypeStr=uint32
  wires:
  PackSubsystem/1(PackOut) -> Convert2BusArray/1(InBus)
  Convert2BusArray/1(BusArrayOut) -> CANWrite/2
  Product/1 -> CANWrite/1
  TxControl/1 -> Product/2
  Enable All/1 -> Product/1
  ID290_AMR_vehicle_speed.speed_m_per_min/1 -> InputSubsystem/1(In1_1)
  ID290_AMR_vehicle_speed.speed_m_per_s/1 -> InputSubsystem/2(In1_2)
  InputSubsystem/1(OutBus) -> PackSubsystem/1(PackIn)

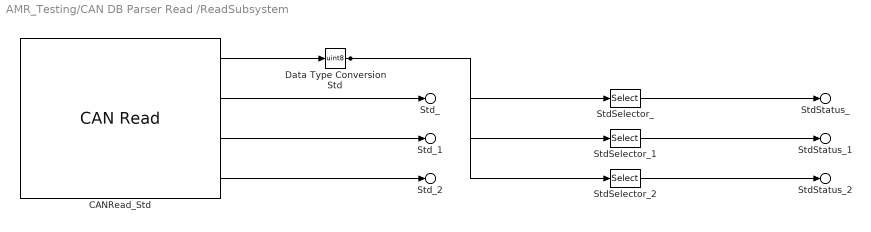
== system AMR_Testing/CAN DB Parser Read /ReadSubsystem ==
  CANRead_Std : speedgoatlib_IO60X_IO69X/CAN/CAN Read   moduleType=IO691  id=1  channel=1  canType=CAN (HS)  messageType=CAN (HS)  useBusOut=on  HasMulRead=Specify by IDs  MsgIDlist="[17  49  52]"  isEFF=off  LabelInHex=off  enableInput=off  initValues=[691 1 0.01 0 1 1 0 1 2 0 3 17 49 52]  ts=10e-3
  Data Type ConversionStd : DataTypeConversion  OutDataTypeStr=uint8  SaturateOnIntegerOverflow=off  RndMeth=Floor
  StdSelector_ : Selector  IndexOptions=Index vector (dialog)  Indices=1  OutputSizes=1
  StdSelector_1 : Selector  IndexOptions=Index vector (dialog)  Indices=2  OutputSizes=1
  StdSelector_2 : Selector  IndexOptions=Index vector (dialog)  Indices=3  OutputSizes=1
  Std_ : Outport  PortName=Raw_Rx  Element=Std.ID17
  Std_1 : Outport  PortName=Raw_Rx  Element=Std.ID49
  Std_2 : Outport  PortName=Raw_Rx  Element=Std.ID52
  StdStatus_ : Outport  Port=2  PortName=Status_Rx  Element=Std.ID17
  StdStatus_1 : Outport  Port=2  PortName=Status_Rx  Element=Std.ID49
  StdStatus_2 : Outport  Port=2  PortName=Status_Rx  Element=Std.ID52
  wires:
  CANRead_Std/1 -> Data Type ConversionStd/1
  CANRead_Std/2 -> Std_/1
  CANRead_Std/3 -> Std_1/1
  CANRead_Std/4 -> Std_2/1
  Data Type ConversionStd/1 -> StdSelector_/1, StdSelector_1/1, StdSelector_2/1
  StdSelector_/1 -> StdStatus_/1
  StdSelector_1/1 -> StdStatus_1/1
  StdSelector_2/1 -> StdStatus_2/1

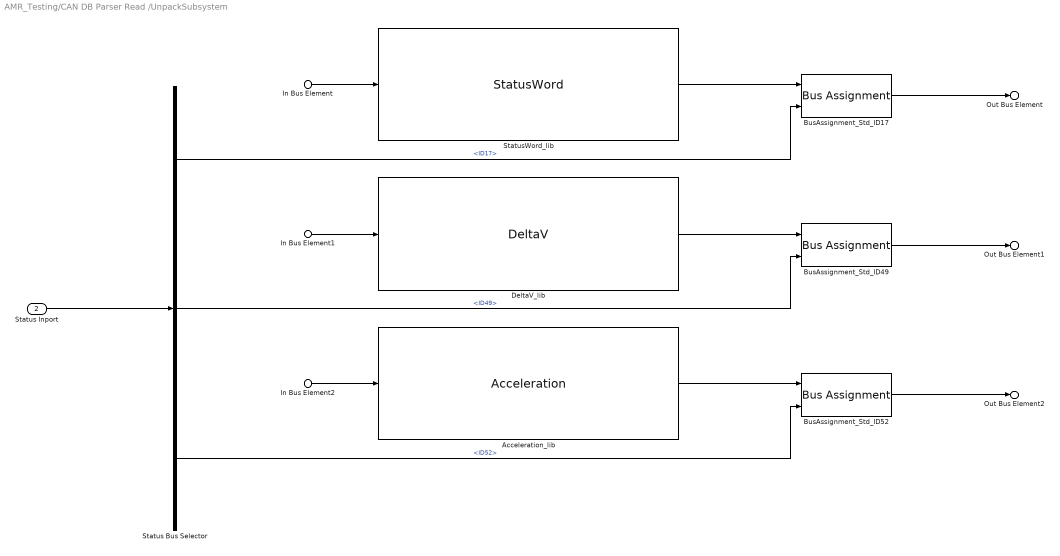
== system AMR_Testing/CAN DB Parser Read /UnpackSubsystem ==
  In Bus Element : Inport  PortName=Unpack_In  Element=Std.ID17
  In Bus Element1 : Inport  PortName=Unpack_In  Element=Std.ID49
  In Bus Element2 : Inport  PortName=Unpack_In  Element=Std.ID52
  Status Inport : Inport  Port=2
  Acceleration_lib : tramontina_database_xsenslib/CAN unpack/Acceleration  SystemSampleTime=-1  VariantActivationTime=update diagram  AllowFlexibleInterface=on  Latency=0  AutoFrameSizeCalculation=off
  BusAssignment_Std_ID17 : BusAssignment  AssignedSignals=MessageStatus.Status
  BusAssignment_Std_ID49 : BusAssignment  AssignedSignals=MessageStatus.Status
  BusAssignment_Std_ID52 : BusAssignment  AssignedSignals=MessageStatus.Status
  DeltaV_lib : tramontina_database_xsenslib/CAN unpack/DeltaV  SystemSampleTime=-1  VariantActivationTime=update diagram  AllowFlexibleInterface=on  Latency=0  AutoFrameSizeCalculation=off
  Status Bus Selector : BusSelector  OutputSignals=Std.ID17,Std.ID49,Std.ID52
  StatusWord_lib : tramontina_database_xsenslib/CAN unpack/StatusWord  SystemSampleTime=-1  VariantActivationTime=update diagram  AllowFlexibleInterface=on  Latency=0  AutoFrameSizeCalculation=off
  Out Bus Element : Outport  PortName=Unpack_Out  Element=ID17_StatusWord
  Out Bus Element1 : Outport  PortName=Unpack_Out  Element=ID49_DeltaV
  Out Bus Element2 : Outport  PortName=Unpack_Out  Element=ID52_Acceleration
  wires:
  In Bus Element/1 -> StatusWord_lib/1
  StatusWord_lib/1 -> BusAssignment_Std_ID17/1
  BusAssignment_Std_ID17/1 -> Out Bus Element/1
  In Bus Element1/1 -> DeltaV_lib/1
  DeltaV_lib/1 -> BusAssignment_Std_ID49/1
  BusAssignment_Std_ID49/1 -> Out Bus Element1/1
  In Bus Element2/1 -> Acceleration_lib/1
  Acceleration_lib/1 -> BusAssignment_Std_ID52/1
  BusAssignment_Std_ID52/1 -> Out Bus Element2/1
  Status Inport/1 -> Status Bus Selector/1
  Status Bus Selector/1 -> BusAssignment_Std_ID17/2  "<ID17>"
  Status Bus Selector/2 -> BusAssignment_Std_ID49/2  "<ID49>"
  Status Bus Selector/3 -> BusAssignment_Std_ID52/2  "<ID52>"

== system AMR_Testing/CAN DB Parser Read 10/ReadSubsystem ==
  CANRead_Std : speedgoatlib_IO60X_IO69X/CAN/CAN Read   moduleType=IO691  id=1  channel=1  canType=CAN (HS)  messageType=CAN (HS)  useBusOut=on  HasMulRead=Specify by IDs  MsgIDlist="[422  423]"  isEFF=off  LabelInHex=off  enableInput=off  initValues=[691 1 0.05 0 1 1 0 1 2 0 2 422 423]  ts=50e-3
  Data Type ConversionStd : DataTypeConversion  OutDataTypeStr=uint8  SaturateOnIntegerOverflow=off  RndMeth=Floor
  StdSelector_ : Selector  IndexOptions=Index vector (dialog)  Indices=1  OutputSizes=1
  StdSelector_1 : Selector  IndexOptions=Index vector (dialog)  Indices=2  OutputSizes=1
  Std_ : Outport  PortName=Raw_Rx  Element=Std.ID422
  Std_1 : Outport  PortName=Raw_Rx  Element=Std.ID423
  StdStatus_ : Outport  Port=2  PortName=Status_Rx  Element=Std.ID422
  StdStatus_1 : Outport  Port=2  PortName=Status_Rx  Element=Std.ID423
  wires:
  CANRead_Std/1 -> Data Type ConversionStd/1
  CANRead_Std/2 -> Std_/1
  CANRead_Std/3 -> Std_1/1
  Data Type ConversionStd/1 -> StdSelector_/1, StdSelector_1/1
  StdSelector_/1 -> StdStatus_/1
  StdSelector_1/1 -> StdStatus_1/1

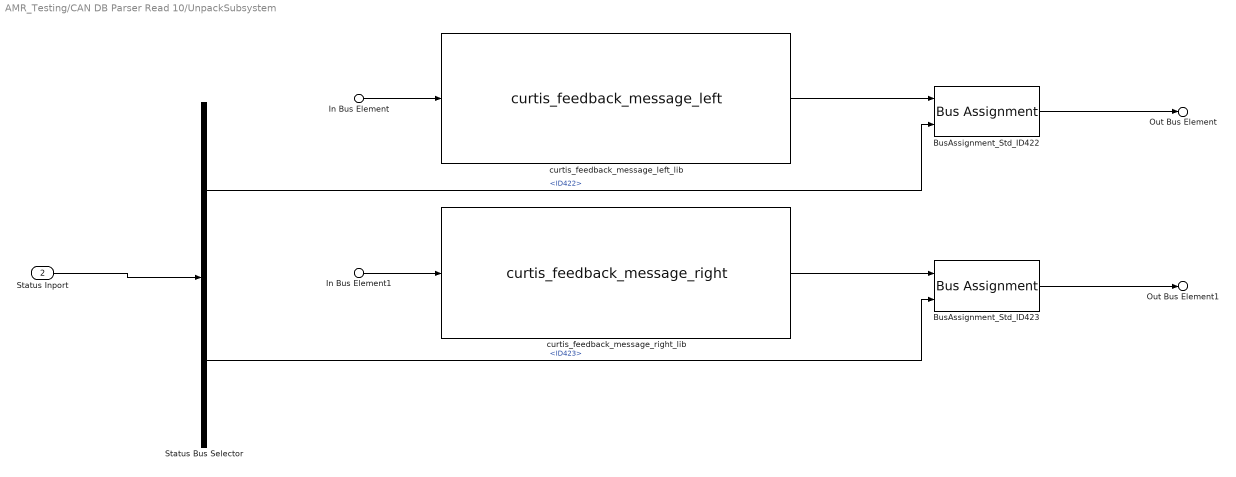
== system AMR_Testing/CAN DB Parser Read 10/UnpackSubsystem ==
  In Bus Element : Inport  PortName=Unpack_In  Element=Std.ID422
  In Bus Element1 : Inport  PortName=Unpack_In  Element=Std.ID423
  Status Inport : Inport  Port=2
  BusAssignment_Std_ID422 : BusAssignment  AssignedSignals=MessageStatus.Status
  BusAssignment_Std_ID423 : BusAssignment  AssignedSignals=MessageStatus.Status
  Status Bus Selector : BusSelector  OutputSignals=Std.ID422,Std.ID423
  curtis_feedback_message_left_lib : tramontina_database_curtislib/CAN unpack/curtis_feedback_message_left  SystemSampleTime=-1  VariantActivationTime=update diagram  AllowFlexibleInterface=on  Latency=0  AutoFrameSizeCalculation=off
  curtis_feedback_message_right_lib : tramontina_database_curtislib/CAN unpack/curtis_feedback_message_right  SystemSampleTime=-1  VariantActivationTime=update diagram  AllowFlexibleInterface=on  Latency=0  AutoFrameSizeCalculation=off
  Out Bus Element : Outport  PortName=Unpack_Out  Element=ID422_curtis_feedback_message_left
  Out Bus Element1 : Outport  PortName=Unpack_Out  Element=ID423_curtis_feedback_message_right
  wires:
  In Bus Element/1 -> curtis_feedback_message_left_lib/1
  curtis_feedback_message_left_lib/1 -> BusAssignment_Std_ID422/1
  BusAssignment_Std_ID422/1 -> Out Bus Element/1
  In Bus Element1/1 -> curtis_feedback_message_right_lib/1
  curtis_feedback_message_right_lib/1 -> BusAssignment_Std_ID423/1
  BusAssignment_Std_ID423/1 -> Out Bus Element1/1
  Status Inport/1 -> Status Bus Selector/1
  Status Bus Selector/1 -> BusAssignment_Std_ID422/2  "<ID422>"
  Status Bus Selector/2 -> BusAssignment_Std_ID423/2  "<ID423>"

== system AMR_Testing/CAN DB Parser Read 11/ReadSubsystem ==
  CANRead_Std : speedgoatlib_IO60X_IO69X/CAN/CAN Read   moduleType=IO691  id=1  channel=1  canType=CAN (HS)  messageType=CAN (HS)  useBusOut=on  HasMulRead=Specify by IDs  MsgIDlist="[1830  1831]"  isEFF=off  LabelInHex=off  enableInput=off  initValues=[691 1 0.5 0 1 1 0 1 2 0 2 1830 1831]  ts=500e-3
  Data Type ConversionStd : DataTypeConversion  OutDataTypeStr=uint8  SaturateOnIntegerOverflow=off  RndMeth=Floor
  StdSelector_ : Selector  IndexOptions=Index vector (dialog)  Indices=1  OutputSizes=1
  StdSelector_1 : Selector  IndexOptions=Index vector (dialog)  Indices=2  OutputSizes=1
  Std_ : Outport  PortName=Raw_Rx  Element=Std.ID1830
  Std_1 : Outport  PortName=Raw_Rx  Element=Std.ID1831
  StdStatus_ : Outport  Port=2  PortName=Status_Rx  Element=Std.ID1830
  StdStatus_1 : Outport  Port=2  PortName=Status_Rx  Element=Std.ID1831
  wires:
  CANRead_Std/1 -> Data Type ConversionStd/1
  CANRead_Std/2 -> Std_/1
  CANRead_Std/3 -> Std_1/1
  Data Type ConversionStd/1 -> StdSelector_/1, StdSelector_1/1
  StdSelector_/1 -> StdStatus_/1
  StdSelector_1/1 -> StdStatus_1/1

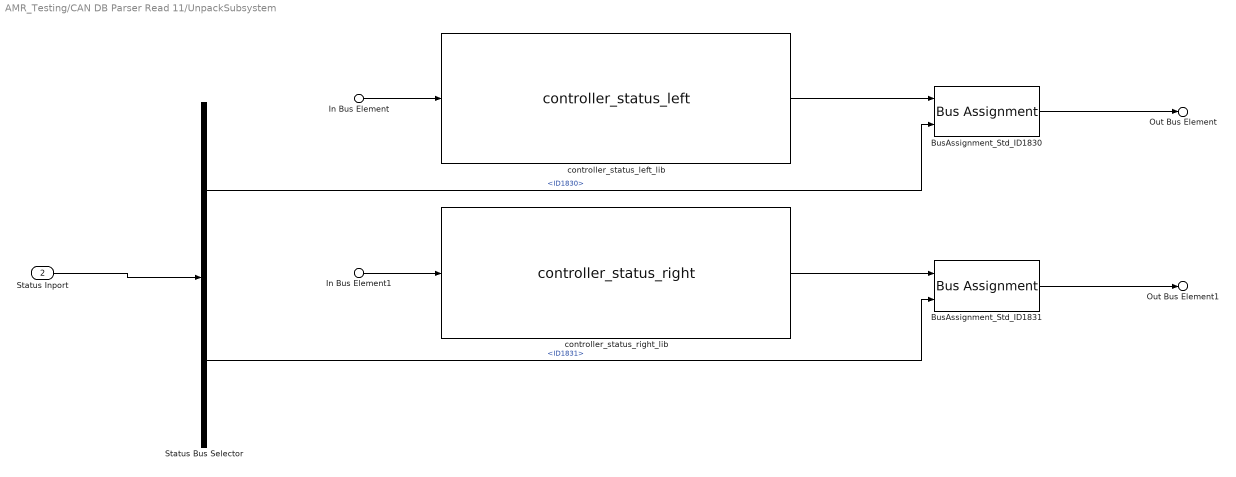
== system AMR_Testing/CAN DB Parser Read 11/UnpackSubsystem ==
  In Bus Element : Inport  PortName=Unpack_In  Element=Std.ID1830
  In Bus Element1 : Inport  PortName=Unpack_In  Element=Std.ID1831
  Status Inport : Inport  Port=2
  BusAssignment_Std_ID1830 : BusAssignment  AssignedSignals=MessageStatus.Status
  BusAssignment_Std_ID1831 : BusAssignment  AssignedSignals=MessageStatus.Status
  Status Bus Selector : BusSelector  OutputSignals=Std.ID1830,Std.ID1831
  controller_status_left_lib : tramontina_database_curtislib/CAN unpack/controller_status_left  SystemSampleTime=-1  VariantActivationTime=update diagram  AllowFlexibleInterface=on  Latency=0  AutoFrameSizeCalculation=off
  controller_status_right_lib : tramontina_database_curtislib/CAN unpack/controller_status_right  SystemSampleTime=-1  VariantActivationTime=update diagram  AllowFlexibleInterface=on  Latency=0  AutoFrameSizeCalculation=off
  Out Bus Element : Outport  PortName=Unpack_Out  Element=ID1830_controller_status_left
  Out Bus Element1 : Outport  PortName=Unpack_Out  Element=ID1831_controller_status_right
  wires:
  In Bus Element/1 -> controller_status_left_lib/1
  controller_status_left_lib/1 -> BusAssignment_Std_ID1830/1
  BusAssignment_Std_ID1830/1 -> Out Bus Element/1
  In Bus Element1/1 -> controller_status_right_lib/1
  controller_status_right_lib/1 -> BusAssignment_Std_ID1831/1
  BusAssignment_Std_ID1831/1 -> Out Bus Element1/1
  Status Inport/1 -> Status Bus Selector/1
  Status Bus Selector/1 -> BusAssignment_Std_ID1830/2  "<ID1830>"
  Status Bus Selector/2 -> BusAssignment_Std_ID1831/2  "<ID1831>"

== system AMR_Testing/CAN DB Parser Read 12/ReadSubsystem ==
  CANRead_Std : speedgoatlib_IO60X_IO69X/CAN/CAN Read   moduleType=IO691  id=1  channel=1  canType=CAN (HS)  messageType=CAN (HS)  useBusOut=on  HasMulRead=Specify by IDs  MsgIDlist="[368  369]"  isEFF=off  LabelInHex=off  enableInput=off  initValues=[691 1 0.01 0 1 1 0 1 2 0 2 368 369]  ts=10e-3
  Data Type ConversionStd : DataTypeConversion  OutDataTypeStr=uint8  SaturateOnIntegerOverflow=off  RndMeth=Floor
  StdSelector_ : Selector  IndexOptions=Index vector (dialog)  Indices=1  OutputSizes=1
  StdSelector_1 : Selector  IndexOptions=Index vector (dialog)  Indices=2  OutputSizes=1
  Std_ : Outport  PortName=Raw_Rx  Element=Std.ID368
  Std_1 : Outport  PortName=Raw_Rx  Element=Std.ID369
  StdStatus_ : Outport  Port=2  PortName=Status_Rx  Element=Std.ID368
  StdStatus_1 : Outport  Port=2  PortName=Status_Rx  Element=Std.ID369
  wires:
  CANRead_Std/1 -> Data Type ConversionStd/1
  CANRead_Std/2 -> Std_/1
  CANRead_Std/3 -> Std_1/1
  Data Type ConversionStd/1 -> StdSelector_/1, StdSelector_1/1
  StdSelector_/1 -> StdStatus_/1
  StdSelector_1/1 -> StdStatus_1/1

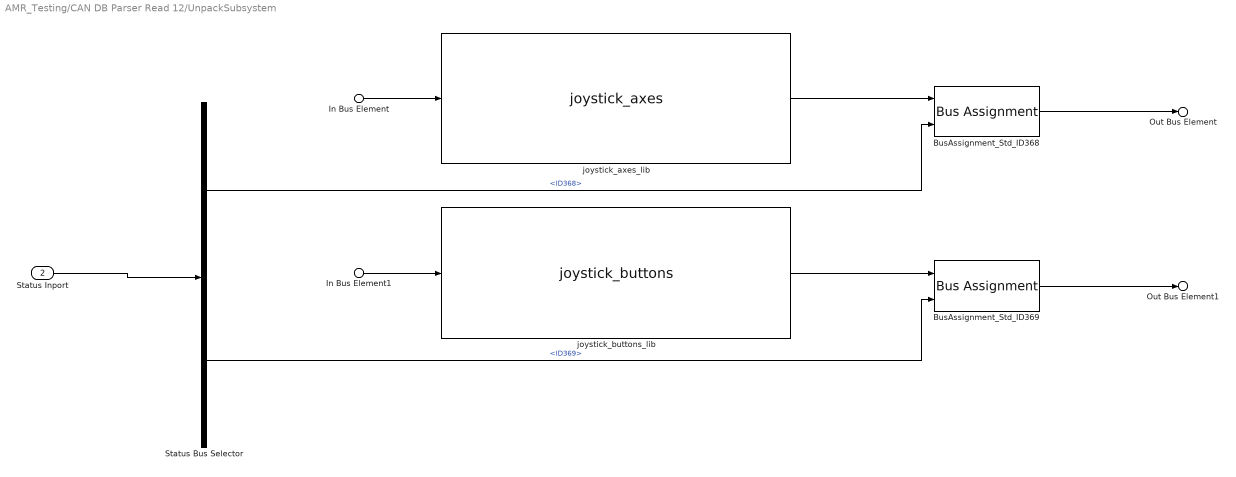
== system AMR_Testing/CAN DB Parser Read 12/UnpackSubsystem ==
  In Bus Element : Inport  PortName=Unpack_In  Element=Std.ID368
  In Bus Element1 : Inport  PortName=Unpack_In  Element=Std.ID369
  Status Inport : Inport  Port=2
  BusAssignment_Std_ID368 : BusAssignment  AssignedSignals=MessageStatus.Status
  BusAssignment_Std_ID369 : BusAssignment  AssignedSignals=MessageStatus.Status
  Status Bus Selector : BusSelector  OutputSignals=Std.ID368,Std.ID369
  joystick_axes_lib : tramontina_database_nvidialib/CAN unpack/joystick_axes  SystemSampleTime=-1  VariantActivationTime=update diagram  AllowFlexibleInterface=on  Latency=0  AutoFrameSizeCalculation=off
  joystick_buttons_lib : tramontina_database_nvidialib/CAN unpack/joystick_buttons  SystemSampleTime=-1  VariantActivationTime=update diagram  AllowFlexibleInterface=on  Latency=0  AutoFrameSizeCalculation=off
  Out Bus Element : Outport  PortName=Unpack_Out  Element=ID368_joystick_axes
  Out Bus Element1 : Outport  PortName=Unpack_Out  Element=ID369_joystick_buttons
  wires:
  In Bus Element/1 -> joystick_axes_lib/1
  joystick_axes_lib/1 -> BusAssignment_Std_ID368/1
  BusAssignment_Std_ID368/1 -> Out Bus Element/1
  In Bus Element1/1 -> joystick_buttons_lib/1
  joystick_buttons_lib/1 -> BusAssignment_Std_ID369/1
  BusAssignment_Std_ID369/1 -> Out Bus Element1/1
  Status Inport/1 -> Status Bus Selector/1
  Status Bus Selector/1 -> BusAssignment_Std_ID368/2  "<ID368>"
  Status Bus Selector/2 -> BusAssignment_Std_ID369/2  "<ID369>"

== system AMR_Testing/CAN DB Parser Read 6/ReadSubsystem ==
  CANRead_Std : speedgoatlib_IO60X_IO69X/CAN/CAN Read   moduleType=IO691  id=1  channel=1  canType=CAN (HS)  messageType=CAN (HS)  useBusOut=on  HasMulRead=Specify by IDs  MsgIDlist="[934  935]"  isEFF=off  LabelInHex=off  enableInput=off  initValues=[691 1 0.01 0 1 1 0 1 2 0 2 934 935]  ts=10e-3
  Data Type ConversionStd : DataTypeConversion  OutDataTypeStr=uint8  SaturateOnIntegerOverflow=off  RndMeth=Floor
  StdSelector_ : Selector  IndexOptions=Index vector (dialog)  Indices=1  OutputSizes=1
  StdSelector_1 : Selector  IndexOptions=Index vector (dialog)  Indices=2  OutputSizes=1
  Std_ : Outport  PortName=Raw_Rx  Element=Std.ID934
  Std_1 : Outport  PortName=Raw_Rx  Element=Std.ID935
  StdStatus_ : Outport  Port=2  PortName=Status_Rx  Element=Std.ID934
  StdStatus_1 : Outport  Port=2  PortName=Status_Rx  Element=Std.ID935
  wires:
  CANRead_Std/1 -> Data Type ConversionStd/1
  CANRead_Std/2 -> Std_/1
  CANRead_Std/3 -> Std_1/1
  Data Type ConversionStd/1 -> StdSelector_/1, StdSelector_1/1
  StdSelector_/1 -> StdStatus_/1
  StdSelector_1/1 -> StdStatus_1/1

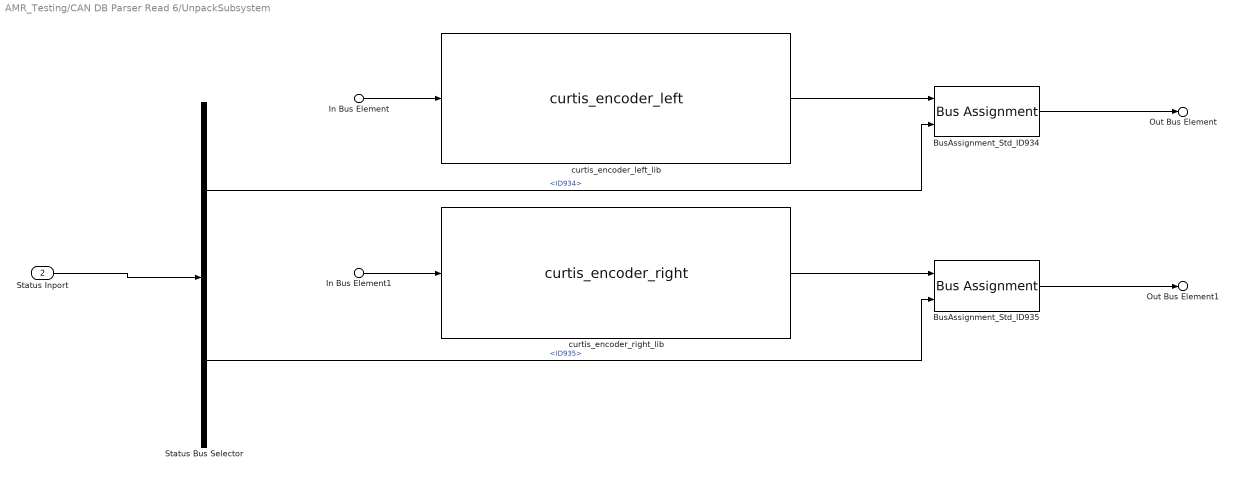
== system AMR_Testing/CAN DB Parser Read 6/UnpackSubsystem ==
  In Bus Element : Inport  PortName=Unpack_In  Element=Std.ID934
  In Bus Element1 : Inport  PortName=Unpack_In  Element=Std.ID935
  Status Inport : Inport  Port=2
  BusAssignment_Std_ID934 : BusAssignment  AssignedSignals=MessageStatus.Status
  BusAssignment_Std_ID935 : BusAssignment  AssignedSignals=MessageStatus.Status
  Status Bus Selector : BusSelector  OutputSignals=Std.ID934,Std.ID935
  curtis_encoder_left_lib : tramontina_database_curtislib/CAN unpack/curtis_encoder_left  SystemSampleTime=-1  VariantActivationTime=update diagram  AllowFlexibleInterface=on  Latency=0  AutoFrameSizeCalculation=off
  curtis_encoder_right_lib : tramontina_database_curtislib/CAN unpack/curtis_encoder_right  SystemSampleTime=-1  VariantActivationTime=update diagram  AllowFlexibleInterface=on  Latency=0  AutoFrameSizeCalculation=off
  Out Bus Element : Outport  PortName=Unpack_Out  Element=ID934_curtis_encoder_left
  Out Bus Element1 : Outport  PortName=Unpack_Out  Element=ID935_curtis_encoder_right
  wires:
  In Bus Element/1 -> curtis_encoder_left_lib/1
  curtis_encoder_left_lib/1 -> BusAssignment_Std_ID934/1
  BusAssignment_Std_ID934/1 -> Out Bus Element/1
  In Bus Element1/1 -> curtis_encoder_right_lib/1
  curtis_encoder_right_lib/1 -> BusAssignment_Std_ID935/1
  BusAssignment_Std_ID935/1 -> Out Bus Element1/1
  Status Inport/1 -> Status Bus Selector/1
  Status Bus Selector/1 -> BusAssignment_Std_ID934/2  "<ID934>"
  Status Bus Selector/2 -> BusAssignment_Std_ID935/2  "<ID935>"

== system AMR_Testing/CAN DB Parser Read 7/ReadSubsystem ==
  CANRead_Std : speedgoatlib_IO60X_IO69X/CAN/CAN Read   moduleType=IO691  id=1  channel=1  canType=CAN (HS)  messageType=CAN (HS)  useBusOut=on  HasMulRead=Specify by IDs  MsgIDlist="[934  935]"  isEFF=off  LabelInHex=off  enableInput=off  initValues=[691 1 0.01 0 1 1 0 1 2 0 2 934 935]  ts=10e-3
  Data Type ConversionStd : DataTypeConversion  OutDataTypeStr=uint8  SaturateOnIntegerOverflow=off  RndMeth=Floor
  StdSelector_ : Selector  IndexOptions=Index vector (dialog)  Indices=1  OutputSizes=1
  StdSelector_1 : Selector  IndexOptions=Index vector (dialog)  Indices=2  OutputSizes=1
  Std_ : Outport  PortName=Raw_Rx  Element=Std.ID934
  Std_1 : Outport  PortName=Raw_Rx  Element=Std.ID935
  StdStatus_ : Outport  Port=2  PortName=Status_Rx  Element=Std.ID934
  StdStatus_1 : Outport  Port=2  PortName=Status_Rx  Element=Std.ID935
  wires:
  StdSelector_1/1 -> StdStatus_1/1
  StdSelector_/1 -> StdStatus_/1
  Data Type ConversionStd/1 -> StdSelector_1/1, StdSelector_/1
  CANRead_Std/3 -> Std_1/1
  CANRead_Std/2 -> Std_/1
  CANRead_Std/1 -> Data Type ConversionStd/1
